simulink model "Panchito_Modelado"  (R2026b)
settings: Solver=VariableStepAuto
settings Model: Creator=david  LastModifiedBy=david

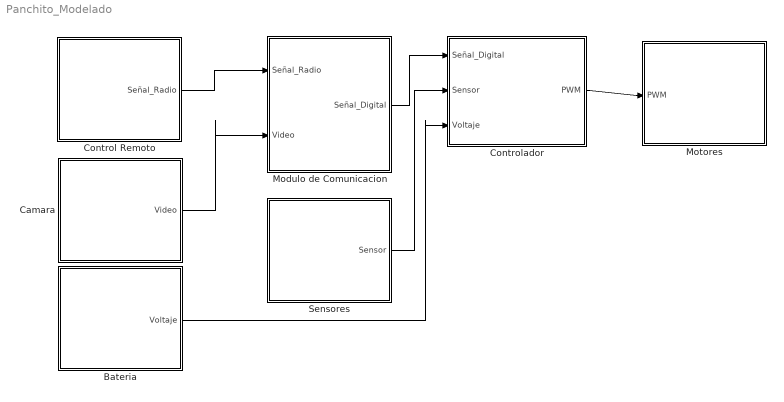
== system Panchito_Modelado ==
  Bateria : Subsystem
      settings: PortSchema="{\"entries\":[{\"content\":{\"headerSize\":26,\"margin\":15,\"minimumSpacing\":25,\"sides\":[{\"content\":{},\"type\":\"ConnectorPlacement.EquallySpacedRectSide\",\"uuid\":\"396280ee-0207-478e-a623-32d0cc6f5b5a\"},{\"content\":{\"connectorIds\":[\"Out1\"],\"side\":\"RIGHT\"},\"type\":\"ConnectorPlacement.EquallySpacedRectSide\",\"uuid\":\"8359d95d-4977-4d96-aead-9dff78753e61\"},{\"content\":{\"side\":\"TOP\"},\"type\":\"ConnectorPlacement.EquallySpacedRectSide\",\"uuid\":\"b2e274a3-0e25-42d5-8b5e-7ee5ddcabd81\"}]},\"type\":\"ConnectorPlacement.EquallySpacedConnector\",\"uuid\":\"a4f514dd-fd39-48ce-9569-33d30d804466\"}],\"packageUris\":[\"http://schema.mathworks.com/mf0/Connector/R2020b\"],\"version\":\"1.0\"}"
  Camara : Subsystem
      settings: PortSchema="{\"entries\":[{\"content\":{\"headerSize\":26,\"margin\":15,\"minimumSpacing\":25,\"sides\":[{\"content\":{},\"type\":\"ConnectorPlacement.EquallySpacedRectSide\",\"uuid\":\"396280ee-0207-478e-a623-32d0cc6f5b5a\"},{\"content\":{\"connectorIds\":[\"Out1\"],\"side\":\"RIGHT\"},\"type\":\"ConnectorPlacement.EquallySpacedRectSide\",\"uuid\":\"8359d95d-4977-4d96-aead-9dff78753e61\"},{\"content\":{\"side\":\"TOP\"},\"type\":\"ConnectorPlacement.EquallySpacedRectSide\",\"uuid\":\"b2e274a3-0e25-42d5-8b5e-7ee5ddcabd81\"}]},\"type\":\"ConnectorPlacement.EquallySpacedConnector\",\"uuid\":\"a4f514dd-fd39-48ce-9569-33d30d804466\"}],\"packageUris\":[\"http://schema.mathworks.com/mf0/Connector/R2020b\"],\"version\":\"1.0\"}"
  Control Remoto : Subsystem
      settings: PortSchema="{\"entries\":[{\"content\":{\"headerSize\":26,\"margin\":15,\"minimumSpacing\":25,\"sides\":[{\"content\":{},\"type\":\"ConnectorPlacement.EquallySpacedRectSide\",\"uuid\":\"396280ee-0207-478e-a623-32d0cc6f5b5a\"},{\"content\":{\"connectorIds\":[\"Out1\"],\"side\":\"RIGHT\"},\"type\":\"ConnectorPlacement.EquallySpacedRectSide\",\"uuid\":\"8359d95d-4977-4d96-aead-9dff78753e61\"},{\"content\":{\"side\":\"TOP\"},\"type\":\"ConnectorPlacement.EquallySpacedRectSide\",\"uuid\":\"b2e274a3-0e25-42d5-8b5e-7ee5ddcabd81\"}]},\"type\":\"ConnectorPlacement.EquallySpacedConnector\",\"uuid\":\"a4f514dd-fd39-48ce-9569-33d30d804466\"}],\"packageUris\":[\"http://schema.mathworks.com/mf0/Connector/R2020b\"],\"version\":\"1.0\"}"
  Controlador : Subsystem
      settings: PortSchema="{\"entries\":[{\"content\":{\"headerSize\":26,\"margin\":15,\"minimumSpacing\":25,\"sides\":[{\"content\":{\"connectorIds\":[\"In1\",\"In3\",\"In2\"]},\"type\":\"ConnectorPlacement.EquallySpacedRectSide\",\"uuid\":\"396280ee-0207-478e-a623-32d0cc6f5b5a\"},{\"content\":{\"connectorIds\":[\"Out1\"],\"side\":\"RIGHT\"},\"type\":\"ConnectorPlacement.EquallySpacedRectSide\",\"uuid\":\"8359d95d-4977-4d96-aead-9dff78753e61\"},{\"content\":{\"side\":\"TOP\"},\"type\":\"ConnectorPlacement.EquallySpacedRectSide\",\"uuid\":\"b2e274a3-0e25-42d5-8b5e-7ee5ddcabd81\"}]},\"type\":\"ConnectorPlacement.EquallySpacedConnector\",\"uuid\":\"a4f514dd-fd39-48ce-9569-33d30d804466\"}],\"packageUris\":[\"http://schema.mathworks.com/mf0/Connector/R2020b\"],\"version\":\"1.0\"}"
  Modulo de Comunicacion : Subsystem
      settings: PortSchema="{\"entries\":[{\"content\":{\"headerSize\":26,\"margin\":15,\"minimumSpacing\":25,\"sides\":[{\"content\":{\"connectorIds\":[\"In1\",\"In2\"]},\"type\":\"ConnectorPlacement.EquallySpacedRectSide\",\"uuid\":\"396280ee-0207-478e-a623-32d0cc6f5b5a\"},{\"content\":{\"connectorIds\":[\"Out1\"],\"side\":\"RIGHT\"},\"type\":\"ConnectorPlacement.EquallySpacedRectSide\",\"uuid\":\"8359d95d-4977-4d96-aead-9dff78753e61\"},{\"content\":{\"side\":\"TOP\"},\"type\":\"ConnectorPlacement.EquallySpacedRectSide\",\"uuid\":\"b2e274a3-0e25-42d5-8b5e-7ee5ddcabd81\"}]},\"type\":\"ConnectorPlacement.EquallySpacedConnector\",\"uuid\":\"a4f514dd-fd39-48ce-9569-33d30d804466\"}],\"packageUris\":[\"http://schema.mathworks.com/mf0/Connector/R2020b\"],\"version\":\"1.0\"}"
  Motores : Subsystem
      settings: PortSchema="{\"entries\":[{\"content\":{\"headerSize\":26,\"margin\":15,\"minimumSpacing\":25,\"sides\":[{\"content\":{\"connectorIds\":[\"In1\"]},\"type\":\"ConnectorPlacement.EquallySpacedRectSide\",\"uuid\":\"396280ee-0207-478e-a623-32d0cc6f5b5a\"},{\"content\":{\"side\":\"RIGHT\"},\"type\":\"ConnectorPlacement.EquallySpacedRectSide\",\"uuid\":\"8359d95d-4977-4d96-aead-9dff78753e61\"},{\"content\":{\"side\":\"TOP\"},\"type\":\"ConnectorPlacement.EquallySpacedRectSide\",\"uuid\":\"b2e274a3-0e25-42d5-8b5e-7ee5ddcabd81\"}]},\"type\":\"ConnectorPlacement.EquallySpacedConnector\",\"uuid\":\"a4f514dd-fd39-48ce-9569-33d30d804466\"}],\"packageUris\":[\"http://schema.mathworks.com/mf0/Connector/R2020b\"],\"version\":\"1.0\"}"
  Sensores : Subsystem
      settings: PortSchema="{\"entries\":[{\"content\":{\"headerSize\":26,\"margin\":15,\"minimumSpacing\":25,\"sides\":[{\"content\":{},\"type\":\"ConnectorPlacement.EquallySpacedRectSide\",\"uuid\":\"396280ee-0207-478e-a623-32d0cc6f5b5a\"},{\"content\":{\"connectorIds\":[\"Out1\"],\"side\":\"RIGHT\"},\"type\":\"ConnectorPlacement.EquallySpacedRectSide\",\"uuid\":\"8359d95d-4977-4d96-aead-9dff78753e61\"},{\"content\":{\"side\":\"TOP\"},\"type\":\"ConnectorPlacement.EquallySpacedRectSide\",\"uuid\":\"b2e274a3-0e25-42d5-8b5e-7ee5ddcabd81\"}]},\"type\":\"ConnectorPlacement.EquallySpacedConnector\",\"uuid\":\"a4f514dd-fd39-48ce-9569-33d30d804466\"}],\"packageUris\":[\"http://schema.mathworks.com/mf0/Connector/R2020b\"],\"version\":\"1.0\"}"
  wires:
  Control Remoto/1(Señal_Radio) -> Modulo de Comunicacion/1(Señal_Radio)
  Bateria/1(Voltaje) -> Controlador/2(Voltaje)
  Controlador/1(PWM) -> Motores/1(PWM)
  Modulo de Comunicacion/1(Señal_Digital) -> Controlador/1(Señal_Digital)
  Camara/1(Video) -> Modulo de Comunicacion/2(Video)
  Sensores/1(Sensor) -> Controlador/3(Sensor)

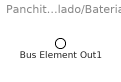
== system Panchito_Modelado/Bateria ==
  Bus Element Out1 : Outport  PortName=Voltaje

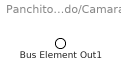
== system Panchito_Modelado/Camara ==
  Bus Element Out1 : Outport  PortName=Video

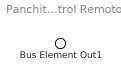
== system Panchito_Modelado/Control Remoto ==
  Bus Element Out1 : Outport  PortName=Señal_Radio

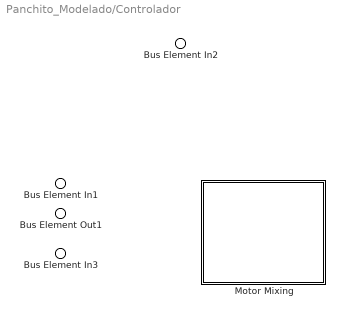
== system Panchito_Modelado/Controlador ==
  Bus Element In2 : Inport  PortName=Señal_Digital
  Bus Element In1 : Inport  Port=2  PortName=Voltaje
  Bus Element In3 : Inport  Port=3  PortName=Sensor
  Motor Mixing : Subsystem
      settings: PortSchema="{\"entries\":[{\"content\":{\"headerSize\":26,\"margin\":15,\"minimumSpacing\":25,\"sides\":[{\"content\":{},\"type\":\"ConnectorPlacement.EquallySpacedRectSide\",\"uuid\":\"396280ee-0207-478e-a623-32d0cc6f5b5a\"},{\"content\":{\"side\":\"RIGHT\"},\"type\":\"ConnectorPlacement.EquallySpacedRectSide\",\"uuid\":\"8359d95d-4977-4d96-aead-9dff78753e61\"},{\"content\":{\"side\":\"TOP\"},\"type\":\"ConnectorPlacement.EquallySpacedRectSide\",\"uuid\":\"b2e274a3-0e25-42d5-8b5e-7ee5ddcabd81\"}]},\"type\":\"ConnectorPlacement.EquallySpacedConnector\",\"uuid\":\"a4f514dd-fd39-48ce-9569-33d30d804466\"}],\"packageUris\":[\"http://schema.mathworks.com/mf0/Connector/R2020b\"],\"version\":\"1.0\"}"
  Bus Element Out1 : Outport  PortName=PWM

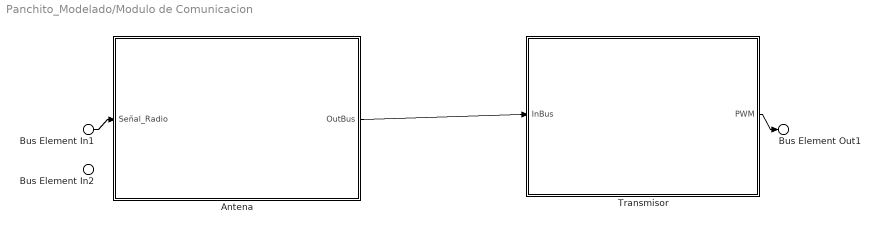
== system Panchito_Modelado/Modulo de Comunicacion ==
  Bus Element In1 : Inport  PortName=Señal_Radio
  Bus Element In2 : Inport  Port=2  PortName=Video
  Antena : Subsystem
      settings: PortSchema="{\"entries\":[{\"content\":{\"headerSize\":26,\"margin\":15,\"minimumSpacing\":25,\"sides\":[{\"content\":{\"connectorIds\":[\"In1\"]},\"type\":\"ConnectorPlacement.EquallySpacedRectSide\",\"uuid\":\"396280ee-0207-478e-a623-32d0cc6f5b5a\"},{\"content\":{\"connectorIds\":[\"Out1\"],\"side\":\"RIGHT\"},\"type\":\"ConnectorPlacement.EquallySpacedRectSide\",\"uuid\":\"8359d95d-4977-4d96-aead-9dff78753e61\"},{\"content\":{\"side\":\"TOP\"},\"type\":\"ConnectorPlacement.EquallySpacedRectSide\",\"uuid\":\"b2e274a3-0e25-42d5-8b5e-7ee5ddcabd81\"}]},\"type\":\"ConnectorPlacement.EquallySpacedConnector\",\"uuid\":\"a4f514dd-fd39-48ce-9569-33d30d804466\"}],\"packageUris\":[\"http://schema.mathworks.com/mf0/Connector/R2020b\"],\"version\":\"1.0\"}"
  Transmisor : Subsystem
      settings: PortSchema="{\"entries\":[{\"content\":{\"headerSize\":26,\"margin\":15,\"minimumSpacing\":25,\"sides\":[{\"content\":{\"connectorIds\":[\"In1\"]},\"type\":\"ConnectorPlacement.EquallySpacedRectSide\",\"uuid\":\"396280ee-0207-478e-a623-32d0cc6f5b5a\"},{\"content\":{\"connectorIds\":[\"Out1\"],\"side\":\"RIGHT\"},\"type\":\"ConnectorPlacement.EquallySpacedRectSide\",\"uuid\":\"8359d95d-4977-4d96-aead-9dff78753e61\"},{\"content\":{\"side\":\"TOP\"},\"type\":\"ConnectorPlacement.EquallySpacedRectSide\",\"uuid\":\"b2e274a3-0e25-42d5-8b5e-7ee5ddcabd81\"}]},\"type\":\"ConnectorPlacement.EquallySpacedConnector\",\"uuid\":\"a4f514dd-fd39-48ce-9569-33d30d804466\"}],\"packageUris\":[\"http://schema.mathworks.com/mf0/Connector/R2020b\"],\"version\":\"1.0\"}"
  Bus Element Out1 : Outport  PortName=Señal_Digital
  wires:
  Bus Element In1/1 -> Antena/1(Señal_Radio)
  Antena/1(OutBus) -> Transmisor/1(InBus)
  Transmisor/1(PWM) -> Bus Element Out1/1

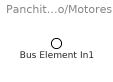
== system Panchito_Modelado/Motores ==
  Bus Element In1 : Inport  PortName=PWM

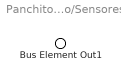
== system Panchito_Modelado/Sensores ==
  Bus Element Out1 : Outport  PortName=Sensor

== system Panchito_Modelado/Controlador/Motor Mixing ==

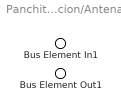
== system Panchito_Modelado/Modulo de Comunicacion/Antena ==
  Bus Element In1 : Inport  PortName=Señal_Radio
  Bus Element Out1 : Outport  PortName=OutBus

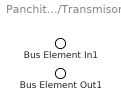
== system Panchito_Modelado/Modulo de Comunicacion/Transmisor ==
  Bus Element In1 : Inport  PortName=InBus
  Bus Element Out1 : Outport  PortName=PWM
